simulink model "OnBoardOk_Computer"  (R2015b)
settings: Solver=VariableStepAuto  StartTime=0.0  StopTime=inf  RelTol=1e-3
libraries: amg_usbconverter_n_connect_lib x1
settings Model: Creator=Hi  LastModifiedBy=Jasper Gundersen

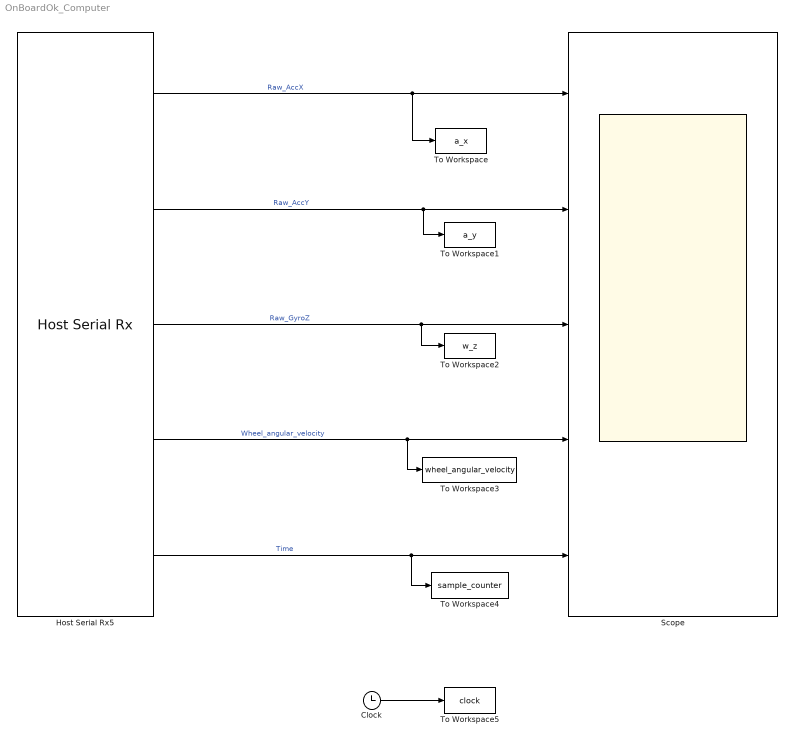
== system OnBoardOk_Computer ==
  Clock : Clock
  Host Serial Rx5 : amg_usbconverter_n_connect_lib/Host Serial Rx  conf=rx  port=COM4  baudrate=115200  databits=8  parity=None  stopbit=1  flowcontrol=None  transfer=Blocking  timeout=5  packetmode=Binary  enableinitialvalues=off  initialvalues=[]  binheader='0E 0E'  binterminator='0A 0A'  porttype_double=5  porttype_single=0  porttype_int8=0  porttype_uint8=0  porttype_int16=0  porttype_uint16=0  porttype_int32=0  porttype_uint32=0  asciiformat='OutX=%d,OutY=%d,OutZ=%d'  rx_asciiterminator="CRLF (0x0D 0x0A - \"\\r\\n\")"  tx_asciiterminator="CRLF (0x0D 0x0A - \"\\r\\n\")"  sampletime=0.002  enablecustomportlabel=off  cinputportlabel=0  coutputportlabel=A  portpinstr=0  blockid=HostSerialRx5  inputporttype=[]  inputportwidth=[]  inputportlabel={}  outputporttype=[0 0 0 0 0]  outputportwidth=[1 1 1 1 1]  outputportlabel={'double','double','double','double','double'}  compat=0  optionstring=[]  autoport='COM4'
  Scope : Scope  NumInputPorts=5
  To Workspace : ToWorkspace  VariableName=a_x  SaveFormat=Timeseries  SampleTime=-1
  To Workspace1 : ToWorkspace  VariableName=a_y  SaveFormat=Timeseries  SampleTime=-1
  To Workspace2 : ToWorkspace  VariableName=w_z  SaveFormat=Timeseries  SampleTime=-1
  To Workspace3 : ToWorkspace  VariableName=wheel_angular_velocity  SaveFormat=Timeseries  SampleTime=-1
  To Workspace4 : ToWorkspace  VariableName=sample_counter  SaveFormat=Timeseries  SampleTime=-1
  To Workspace5 : ToWorkspace  VariableName=clock  SaveFormat=Timeseries  SampleTime=-1
  wires:
  Host Serial Rx5/1 -> To Workspace/1, Scope/1  "Raw_AccX"
  Host Serial Rx5/2 -> To Workspace1/1, Scope/2  "Raw_AccY"
  Host Serial Rx5/3 -> To Workspace2/1, Scope/3  "Raw_GyroZ"
  Host Serial Rx5/4 -> To Workspace3/1, Scope/4  "Wheel_angular_velocity"
  Host Serial Rx5/5 -> To Workspace4/1, Scope/5  "Time"
  Clock/1 -> To Workspace5/1
